simulink model "Test_Byte_Multiplexer_16_to_1"  (Simulink 8.1)
settings: Solver=ode45  StartTime=0.0  StopTime=len  RelTol=1e-3
libraries: Byte_Multiplexers_Lib x1, commutil2 x1
settings Model: Creator=N  LastModifiedBy=uzivatel
settings DataIOCC: LimitDataPoints=off  SignalLoggingSaveFormat=Dataset
settings OptimizationCC: ExpressionDepthLimit=128
settings DebuggingCC: UnderspecifiedInitializationDetection=Simplified  MergeDetectMultiDrivingBlocksExec=error  SolverPrmCheckMsg=none  FcnCallInpInsideContextMsg=EnableAllAsError  FrameProcessingCompatibilityMsg=error  StateNameClashWarn=none
settings HardwareCC: ProdBitPerPointer=64  ProdLargestAtomicFloat=Float  ProdIntDivRoundTo=Zero  ProdEndianess=LittleEndian  ProdHWDeviceType=Intel->x86-64 (Windows64)
settings ModelReferenceCC: PropagateSignalLabelsOutOfModel=on
settings GRTTargetCC: CodeReplacementLibrary=None  CombineOutputUpdateFcns=on  CPPClassGenCompliant=on  GRTInterface=off

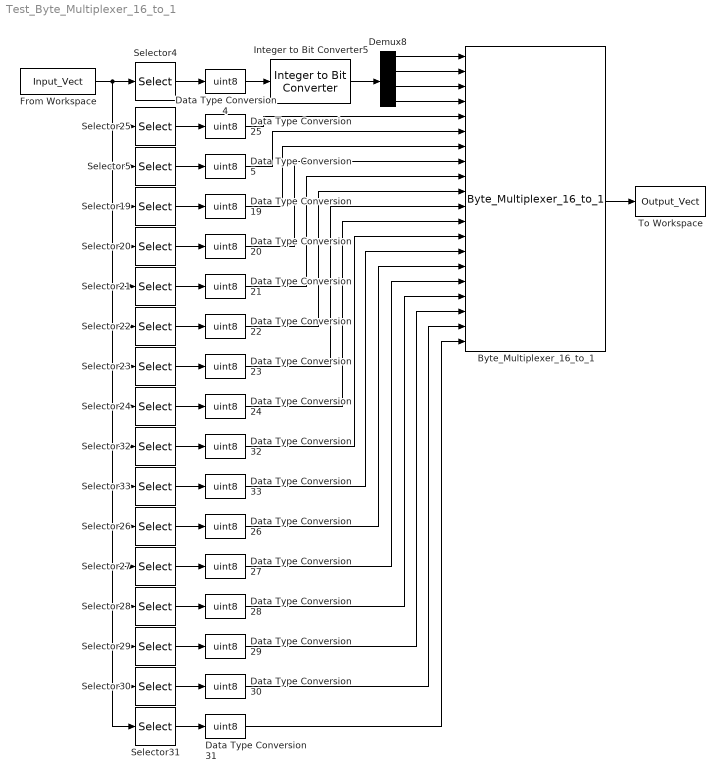
== system Test_Byte_Multiplexer_16_to_1 ==
  Byte_Multiplexer_16_to_1 : Byte_Multiplexers_Lib/Byte_Multiplexers_Lib/Byte_Multiplexer_16_to_1
  Data Type Conversion{4..5,19..33} (17 alike) : DataTypeConversion  OutDataTypeStr=uint8
  Demux8 : Demux
  From Workspace : FromWorkspace  VariableName=Input_Vect  SampleTime=1  Interpolate=off  OutputAfterFinalValue=Holding final value
  Integer to Bit Converter5 : commutil2/Integer to Bit Converter  nbits=4  signedInputValues=Unsigned  bitOrder=MSB first  outDtype=boolean
  Selector19 : Selector  IndexMode=Zero-based  InputPortWidth=17  IndexOptions=Index vector (dialog)  Indices=3  OutputSizes=1
  Selector20 : Selector  IndexMode=Zero-based  InputPortWidth=17  IndexOptions=Index vector (dialog)  Indices=4  OutputSizes=1
  Selector21 : Selector  IndexMode=Zero-based  InputPortWidth=17  IndexOptions=Index vector (dialog)  Indices=5  OutputSizes=1
  Selector22 : Selector  IndexMode=Zero-based  InputPortWidth=17  IndexOptions=Index vector (dialog)  Indices=6  OutputSizes=1
  Selector23 : Selector  IndexMode=Zero-based  InputPortWidth=17  IndexOptions=Index vector (dialog)  Indices=7  OutputSizes=1
  Selector24 : Selector  IndexMode=Zero-based  InputPortWidth=17  IndexOptions=Index vector (dialog)  Indices=8  OutputSizes=1
  Selector25 : Selector  IndexMode=Zero-based  InputPortWidth=17  IndexOptions=Index vector (dialog)  Indices=1  OutputSizes=1
  Selector26 : Selector  IndexMode=Zero-based  InputPortWidth=17  IndexOptions=Index vector (dialog)  Indices=11  OutputSizes=1
  Selector27 : Selector  IndexMode=Zero-based  InputPortWidth=17  IndexOptions=Index vector (dialog)  Indices=12  OutputSizes=1
  Selector28 : Selector  IndexMode=Zero-based  InputPortWidth=17  IndexOptions=Index vector (dialog)  Indices=13  OutputSizes=1
  Selector29 : Selector  IndexMode=Zero-based  InputPortWidth=17  IndexOptions=Index vector (dialog)  Indices=14  OutputSizes=1
  Selector30 : Selector  IndexMode=Zero-based  InputPortWidth=17  IndexOptions=Index vector (dialog)  Indices=15  OutputSizes=1
  Selector31 : Selector  IndexMode=Zero-based  InputPortWidth=17  IndexOptions=Index vector (dialog)  Indices=16  OutputSizes=1
  Selector32 : Selector  IndexMode=Zero-based  InputPortWidth=17  IndexOptions=Index vector (dialog)  Indices=9  OutputSizes=1
  Selector33 : Selector  IndexMode=Zero-based  InputPortWidth=17  IndexOptions=Index vector (dialog)  Indices=10  OutputSizes=1
  Selector4 : Selector  IndexMode=Zero-based  InputPortWidth=17  SampleTime=1  IndexOptions=Index vector (dialog)  Indices=0  OutputSizes=1
  Selector5 : Selector  IndexMode=Zero-based  InputPortWidth=17  IndexOptions=Index vector (dialog)  Indices=2  OutputSizes=1
  To Workspace : ToWorkspace  VariableName=Output_Vect  SampleTime=1
  wires:
  Integer to Bit Converter5/1 -> Demux8/1
  Byte_Multiplexer_16_to_1/1 -> To Workspace/1
  Demux8/1 -> Byte_Multiplexer_16_to_1/1
  Demux8/3 -> Byte_Multiplexer_16_to_1/3
  Demux8/2 -> Byte_Multiplexer_16_to_1/2
  Demux8/4 -> Byte_Multiplexer_16_to_1/4
  Selector4/1 -> Data Type Conversion4/1
  Data Type Conversion4/1 -> Integer to Bit Converter5/1
  From Workspace/1 -> Selector5/1, Selector19/1, Selector20/1, Selector21/1, Selector22/1, Selector23/1, Selector32/1, Selector33/1, Selector26/1, Selector27/1, Selector28/1, Selector29/1, Selector30/1, Selector31/1, Selector24/1, Selector25/1, Selector4/1
  Selector25/1 -> Data Type Conversion25/1
  Data Type Conversion25/1 -> Byte_Multiplexer_16_to_1/5
  Selector5/1 -> Data Type Conversion5/1
  Selector19/1 -> Data Type Conversion19/1
  Selector20/1 -> Data Type Conversion20/1
  Selector21/1 -> Data Type Conversion21/1
  Selector22/1 -> Data Type Conversion22/1
  Selector23/1 -> Data Type Conversion23/1
  Selector24/1 -> Data Type Conversion24/1
  Data Type Conversion5/1 -> Byte_Multiplexer_16_to_1/6
  Data Type Conversion19/1 -> Byte_Multiplexer_16_to_1/7
  Data Type Conversion20/1 -> Byte_Multiplexer_16_to_1/8
  Data Type Conversion21/1 -> Byte_Multiplexer_16_to_1/9
  Data Type Conversion22/1 -> Byte_Multiplexer_16_to_1/10
  Data Type Conversion23/1 -> Byte_Multiplexer_16_to_1/11
  Data Type Conversion24/1 -> Byte_Multiplexer_16_to_1/12
  Selector32/1 -> Data Type Conversion32/1
  Data Type Conversion32/1 -> Byte_Multiplexer_16_to_1/13
  Selector33/1 -> Data Type Conversion33/1
  Selector26/1 -> Data Type Conversion26/1
  Selector27/1 -> Data Type Conversion27/1
  Selector28/1 -> Data Type Conversion28/1
  Selector29/1 -> Data Type Conversion29/1
  Selector30/1 -> Data Type Conversion30/1
  Selector31/1 -> Data Type Conversion31/1
  Data Type Conversion33/1 -> Byte_Multiplexer_16_to_1/14
  Data Type Conversion26/1 -> Byte_Multiplexer_16_to_1/15
  Data Type Conversion27/1 -> Byte_Multiplexer_16_to_1/16
  Data Type Conversion28/1 -> Byte_Multiplexer_16_to_1/17
  Data Type Conversion29/1 -> Byte_Multiplexer_16_to_1/18
  Data Type Conversion30/1 -> Byte_Multiplexer_16_to_1/19
  Data Type Conversion31/1 -> Byte_Multiplexer_16_to_1/20
